simulink model "Cw1"  (R2016b)
settings: Solver=VariableStepDiscrete  StartTime=0.0  StopTime=1e-3  RelTol=1e-3
libraries: dspsrcs4 x2, commchan3 x1, dsparch4 x1, commseqgen3 x1, commutil2 x1
settings Model: Creator=Krzysztof  LastModifiedBy=Krzysztof

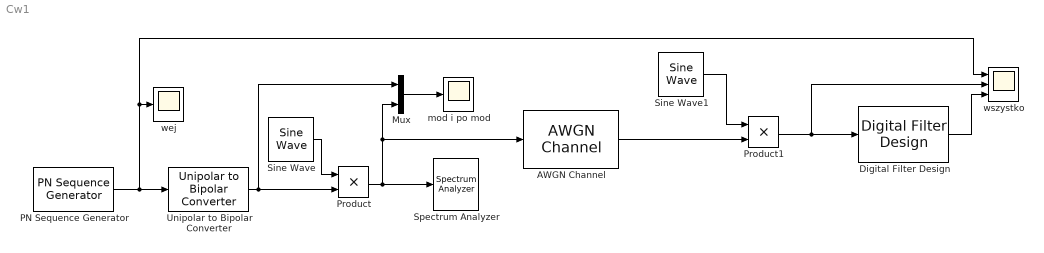
== system Cw1 ==
  AWGN Channel : commchan3/AWGN Channel  InputProcessing=Columns as channels (frame based)  seed=67  noiseMode="Signal to noise ratio  (SNR)"  EbNodB=10  EsNodB=10  SNRdB=30  bitsPerSym=1  Ps=1  Tsym=1  variance=1
  Digital Filter Design : dsparch4/Digital Filter Design  mwdsp_browser_bugfix_var=off
  Mux : Mux  Inputs=2
  PN Sequence Generator : commseqgen3/PN Sequence Generator  poly=[7 6 0]  ini_sta=[0 0 1 0 0 1 0]  outBitMaskSource=Dialog parameter  shift=0  outVarSiz=off  maxOutSizeMode=Dialog parameter  maxOutSize=[10 1]  Ts=1/500e3  sampPerFrame=1  reset=off  bitPackedOutputs=off  outDataType=double  numPackedBits=8  bitPackDataSigned=off  bitPackedOutDType=double
  Product : Product
  Product1 : Product
  Sine Wave : dspsrcs4/Sine Wave  Amplitude=0.9  Frequency=20e6  Phase=0  SampleMode=Discrete  OutComplex=Real  CompMethod=Trigonometric fcn  TableSize=Speed  SampleTime=1/200e6  SamplesPerFrame=1  ResetState=Restart at time zero  OutputFrames=off  dataType=double  wordLen=16  udDataType=sfix(16)  fracBitsMode=Best precision  numFracBits=15  OutDataTypeStr=double  LastOutDataTypeStr=double
  Sine Wave1 : dspsrcs4/Sine Wave  Amplitude=0.9  Frequency=20e6  Phase=0  SampleMode=Discrete  OutComplex=Real  CompMethod=Trigonometric fcn  TableSize=Speed  SampleTime=1/200e6  SamplesPerFrame=1  ResetState=Restart at time zero  OutputFrames=off  dataType=double  wordLen=16  udDataType=sfix(16)  fracBitsMode=Best precision  numFracBits=15  OutDataTypeStr=double  LastOutDataTypeStr=double
  Spectrum Analyzer : SpectrumAnalyzer
  Unipolar to Bipolar Converter : commutil2/Unipolar to Bipolar Converter  M=2  polarity=Positive  dataType=Inherit via internal rule
  mod i po mod : Scope
  wej : Scope
  "wszystko " : Scope  NumInputPorts=3
  wires:
  PN Sequence Generator/1 -> "wszystko "/1, wej/1, Unipolar to Bipolar Converter/1
  Unipolar to Bipolar Converter/1 -> Mux/1, Product/2
  Product/1 -> AWGN Channel/1, Mux/2, Spectrum Analyzer/1
  Sine Wave/1 -> Product/1
  Mux/1 -> mod i po mod/1
  Sine Wave1/1 -> Product1/1
  AWGN Channel/1 -> Product1/2
  Product1/1 -> "wszystko "/2, Digital Filter Design/1
  Digital Filter Design/1 -> "wszystko "/3
